simulink model "PowerSplitDriveUnit_Component_harness_model"  (R2022b)
settings: Solver=daessc  StartTime=0.0  StopTime=100  RelTol=1e-3  AbsTol=1e-3
PreLoadFcn:
  | PowerSplitDriveUnit_Component_harness_setup
undefined symbols (not defined in the file): batteryHighVoltage, Minus, Plus
libraries: fl_lib x15, nesl_utility x14, sdl_lib x2
settings Model: Creator=isaacito  LastModifiedBy=isaacito
settings SolverCC: AutoScaleAbsTol=off  AlgebraicLoopSolver=TrustRegion
settings DataIOCC: DSMLogging=off  ReturnWorkspaceOutputs=off
settings DebuggingCC: UnconnectedInputMsg=warning  UnconnectedOutputMsg=warning  UnconnectedLineMsg=warning  SymbolicDimsDataTypeCodeGenerationDiagnostic=none  SFMachineParentedDataDiag=warning
settings ModelReferenceCC: EnableRefExpFcnMdlSchedulingChecks=on
settings SFSimCC: CustomCodeUndefinedFunction=UseInterfaceOnly
settings RTWCC: DLArmComputeVersion=19.05
settings SimscapeCC: SimscapeLogType=all  SimscapeLogSimulationStatistics=on  SimscapeLogLimitData=off  SimscapeLogDataHistory=10000

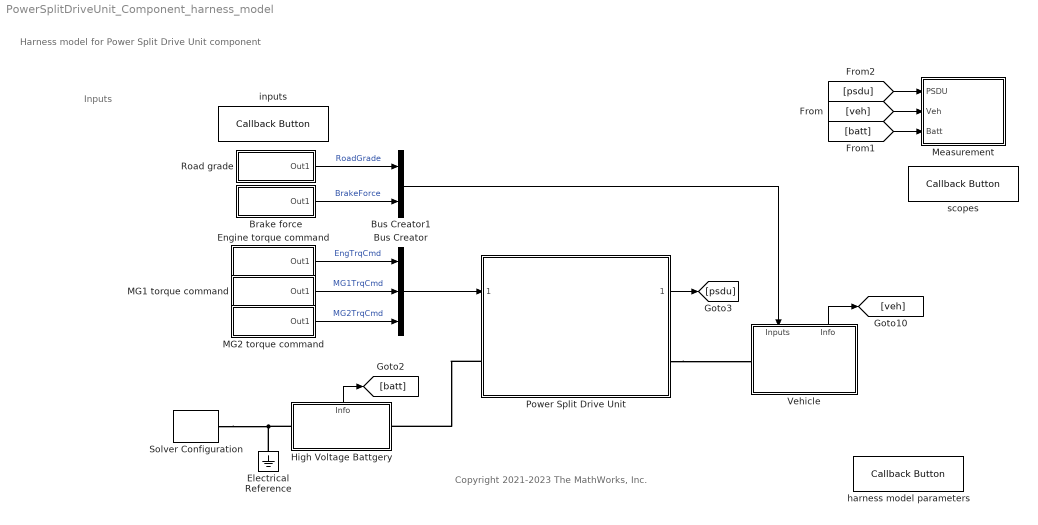
== system PowerSplitDriveUnit_Component_harness_model ==
  note: Inputs
  note: Copyright 2021-2023 The MathWorks, Inc.
  note: Harness model for Power Split Drive Unit component
  Brake force : Subsystem  mask(Continuous Multi-Step Signal){dataPoints=[0 1 0; 2 100 0], deltaT=0.1}
      mask prompts: dataPoints "Data points"; deltaT "Interpolation step [s]"
      mask help:
      | This block generates a signal consisting of smoothly connected flat segments. Data points parameter takes an N-by-3 matrix where each row specifies a flat segment. First column and second column define start and end time of the segment, respectively. Third column defines the value of the segment. Second column can also be NaN to define a point value. Flat segments and point values are smoothly interpolated by Akima spline with the specified interpolation step.
      |
      | For example, a matrix [0 1 5; 3 nan 9; 6 8 7] for Data points defines a signal as follows. First row defines a flat segment from t=0 to t=1 of value 5. Second row defines a point at t=3 of value 9. Third row defines a flat segment from t=6 to t=8 of value 7.
      mask init:
      | sig = SignalDesigner("continuous");
      | 
      | % Initialization function can access parameter names directly
      | sig.XYData = dataPoints;
      | sig.DeltaX = deltaT;
      | 
      | update(sig)
      | 
      | xStr = "[" + num2str(sig.Data.X') + "]";
      | yStr = "[" + num2str(sig.Data.Y') + "]";
      | 
      | set_param([gcb '/1-D Lookup Table'], 'Table', yStr)
      | set_param([gcb '/1-D Lookup Table'], 'BreakpointsForDimension1', xStr)
      mask DialogControl Container3 Prompt: Utility
      mask DialogControl PlotButton Prompt: Plot
      mask DialogControl PlotButton Callback:
      | dataPoints = eval(get_param(gcb, "dataPoints"));
      | deltaT = eval(get_param(gcb, "deltaT"));
      | 
      | sig = SignalDesigner("continuous");
      | sig.DeltaX = deltaT;
      | sig.XYData = dataPoints;
      | sig.XVarName = "Time (s)";
      | sig.YVarName = "Data";
      | update(sig)
      | plotDataPoints(sig);
      mask DialogControl Control3 Prompt: (invisible text area)
      mask Display: disp("Continuous" + newline + "Multi-Step")
  Bus Creator : BusCreator  Inputs=3
  Bus Creator1 : BusCreator  Inputs=2
  Electrical Reference : fl_lib/Electrical/Electrical Elements/Electrical Reference
  Engine torque command : Subsystem  mask(Continuous Multi-Step Signal){dataPoints=[0 13 0; 15 50 80; 52 100 120], deltaT=0.1}
      mask prompts: dataPoints "Data points"; deltaT "Interpolation step [s]"
      mask help:
      | This block generates a signal consisting of smoothly connected flat segments. Data points parameter takes an N-by-3 matrix where each row specifies a flat segment. First column and second column define start and end time of the segment, respectively. Third column defines the value of the segment. Second column can also be NaN to define a point value. Flat segments and point values are smoothly interpolated by Akima spline with the specified interpolation step.
      |
      | For example, a matrix [0 1 5; 3 nan 9; 6 8 7] for Data points defines a signal as follows. First row defines a flat segment from t=0 to t=1 of value 5. Second row defines a point at t=3 of value 9. Third row defines a flat segment from t=6 to t=8 of value 7.
      mask init: same as PowerSplitDriveUnit_Component_harness_model/Brake force
      mask DialogControl Container3 Prompt: Utility
      mask DialogControl PlotButton Prompt: Plot
      mask DialogControl PlotButton Callback:
      | dataPoints = eval(get_param(gcb, "dataPoints"));
      | deltaT = eval(get_param(gcb, "deltaT"));
      | 
      | sig = SignalDesigner("continuous");
      | sig.DeltaX = deltaT;
      | sig.XYData = dataPoints;
      | sig.XVarName = "Time (s)";
      | sig.YVarName = "Data";
      | update(sig)
      | plotDataPoints(sig);
      mask DialogControl Control3 Prompt: (invisible text area)
      mask Display: disp("Continuous" + newline + "Multi-Step")
  High Voltage Battgery : Subsystem
      settings: PortSchema="{\"entries\":[{\"content\":{\"sides\":[{\"content\":{\"connectorIds\":[\"LConn1\"]},\"type\":\"ConnectorPlacement.EquallySpacedRectSide\",\"uuid\":\"8acd7e9a-bb08-4de6-aa14-0989ebba81b9\"},{\"content\":{\"connectorIds\":[\"RConn1\"],\"side\":\"RIGHT\"},\"type\":\"ConnectorPlacement.EquallySpacedRectSide\",\"uuid\":\"f80e1afc-966f-4d6b-84f9-f0b60dd6f20c\"},{\"content\":{\"connectorIds\":[\"Out1\"],\"side\":\"TOP\"},\"type\":\"ConnectorPlacement.EquallySpacedRectSide\",\"uuid\":\"52ccb2b1-bd5e-4dcb-b9b6-0ef03b912c33\"}]},\"type\":\"ConnectorPlacement.EquallySpacedConnector\",\"uuid\":\"b55f48a4-f283-4a77-8513-99b31abb285a\"}],\"packageUris\":[\"http://schema.mathworks.com/mf0/Connector/R2020b\"],\"version\":\"1.0\"}"
  MG1 torque command : Subsystem  mask(Continuous Multi-Step Signal){dataPoints=[0 10 0; 12 15 9; 16 100 0], deltaT=0.1}
      mask prompts: dataPoints "Data points"; deltaT "Interpolation step [s]"
      mask help:
      | This block generates a signal consisting of smoothly connected flat segments. Data points parameter takes an N-by-3 matrix where each row specifies a flat segment. First column and second column define start and end time of the segment, respectively. Third column defines the value of the segment. Second column can also be NaN to define a point value. Flat segments and point values are smoothly interpolated by Akima spline with the specified interpolation step.
      |
      | For example, a matrix [0 1 5; 3 nan 9; 6 8 7] for Data points defines a signal as follows. First row defines a flat segment from t=0 to t=1 of value 5. Second row defines a point at t=3 of value 9. Third row defines a flat segment from t=6 to t=8 of value 7.
      mask init: same as PowerSplitDriveUnit_Component_harness_model/Brake force
      mask DialogControl Container3 Prompt: Utility
      mask DialogControl PlotButton Prompt: Plot
      mask DialogControl PlotButton Callback:
      | dataPoints = eval(get_param(gcb, "dataPoints"));
      | deltaT = eval(get_param(gcb, "deltaT"));
      | 
      | sig = SignalDesigner("continuous");
      | sig.DeltaX = deltaT;
      | sig.XYData = dataPoints;
      | sig.XVarName = "Time (s)";
      | sig.YVarName = "Data";
      | update(sig)
      | plotDataPoints(sig);
      mask DialogControl Control3 Prompt: (invisible text area)
      mask Display: disp("Continuous" + newline + "Multi-Step")
  MG2 torque command : Subsystem  mask(Continuous Multi-Step Signal){dataPoints=[0 1 0; 2 100 0], deltaT=0.1}
      mask prompts: dataPoints "Data points"; deltaT "Interpolation step [s]"
      mask help:
      | This block generates a signal consisting of smoothly connected flat segments. Data points parameter takes an N-by-3 matrix where each row specifies a flat segment. First column and second column define start and end time of the segment, respectively. Third column defines the value of the segment. Second column can also be NaN to define a point value. Flat segments and point values are smoothly interpolated by Akima spline with the specified interpolation step.
      |
      | For example, a matrix [0 1 5; 3 nan 9; 6 8 7] for Data points defines a signal as follows. First row defines a flat segment from t=0 to t=1 of value 5. Second row defines a point at t=3 of value 9. Third row defines a flat segment from t=6 to t=8 of value 7.
      mask init: same as PowerSplitDriveUnit_Component_harness_model/Brake force
      mask DialogControl Container3 Prompt: Utility
      mask DialogControl PlotButton Prompt: Plot
      mask DialogControl PlotButton Callback:
      | dataPoints = eval(get_param(gcb, "dataPoints"));
      | deltaT = eval(get_param(gcb, "deltaT"));
      | 
      | sig = SignalDesigner("continuous");
      | sig.DeltaX = deltaT;
      | sig.XYData = dataPoints;
      | sig.XVarName = "Time (s)";
      | sig.YVarName = "Data";
      | update(sig)
      | plotDataPoints(sig);
      mask DialogControl Control3 Prompt: (invisible text area)
      mask Display: disp("Continuous" + newline + "Multi-Step")
  Measurement : Subsystem
  Power Split Drive Unit : Subsystem  ReferencedSubsystem=PowerSplitDriveUnit_refsub_Basic
  Road grade : Subsystem  mask(Continuous Multi-Step Signal){dataPoints=[0 1 0; 2 100 0], deltaT=0.1}
      mask prompts: dataPoints "Data points"; deltaT "Interpolation step [s]"
      mask help:
      | This block generates a signal consisting of smoothly connected flat segments. Data points parameter takes an N-by-3 matrix where each row specifies a flat segment. First column and second column define start and end time of the segment, respectively. Third column defines the value of the segment. Second column can also be NaN to define a point value. Flat segments and point values are smoothly interpolated by Akima spline with the specified interpolation step.
      |
      | For example, a matrix [0 1 5; 3 nan 9; 6 8 7] for Data points defines a signal as follows. First row defines a flat segment from t=0 to t=1 of value 5. Second row defines a point at t=3 of value 9. Third row defines a flat segment from t=6 to t=8 of value 7.
      mask init: same as PowerSplitDriveUnit_Component_harness_model/Brake force
      mask DialogControl Container3 Prompt: Utility
      mask DialogControl PlotButton Prompt: Plot
      mask DialogControl PlotButton Callback:
      | dataPoints = eval(get_param(gcb, "dataPoints"));
      | deltaT = eval(get_param(gcb, "deltaT"));
      | 
      | sig = SignalDesigner("continuous");
      | sig.DeltaX = deltaT;
      | sig.XYData = dataPoints;
      | sig.XVarName = "Time (s)";
      | sig.YVarName = "Data";
      | update(sig)
      | plotDataPoints(sig);
      mask DialogControl Control3 Prompt: (invisible text area)
      mask Display: disp("Continuous" + newline + "Multi-Step")
  Solver Configuration : nesl_utility/Solver Configuration  PhysicalDomain=network_engine_domain  SubClassName=solver  LeftPortType=input  RightPortType=generic  Tones=[]  Harmonics=[]  SimulateNoise=off  Profile=off  UseLocalSampling=off  EnableSwitchedLinearOptims=on  FrequencyDomain=off  UseCCode=off  RelTol=0.001  AbsTol=1e-06  MinStep=1e-09  ToWorkspace=off  RevertToSquareIcSolve=off  NumHomotopyIterations=100  PhasorMode=off  PhasorModeNumHarmonics=1  ConsistencySolver=NEWTON_FTOL  IndexReductionMethod=DerivativeReplacement  DoDC=off  ResidualTolerance=1e-09  ConsistencyTolSource=GLOBAL  ConsistencyAbsTol=0.001  ConsistencyRelTol=0.001  ConsistencyTolFactor=0.001  UseLocalSolver=off  LocalSolverChoice=NE_BACKWARD_EULER_ADVANCER  ResolveIndetEquations=on  FunctionEvalNumThread=1  LocalSolverSampleTime=0.001  DoFixedCost=off  MaxNonlinIter=3  MaxModeIter=2  ComputeImpulses=off  ImpulseIterations=2  LinearAlgebra=auto  LinearAlgebraNumThread=0  EquationFormulation=NE_TIME_EF  DelaysMemoryBudget=1024  AutomaticFiltering=on  FilteringTimeConstant=0.001  PartitionStorageMethod=AS_NEEDED  PartitionMemoryBudget=1024  PartitionMethod=ROBUST
      settings: AttributesFormatString=Local solver %<UseLocalSolver>
  Vehicle : Subsystem
      settings: PortSchema="{\"entries\":[{\"content\":{\"sides\":[{\"content\":{\"connectorIds\":[\"LConn1\"]},\"type\":\"ConnectorPlacement.EquallySpacedRectSide\",\"uuid\":\"26173f4b-7c8a-4f16-9397-bd2703a262c3\"},{\"content\":{\"connectorIds\":[],\"side\":\"RIGHT\"},\"type\":\"ConnectorPlacement.EquallySpacedRectSide\",\"uuid\":\"c1cca5f5-e160-4db7-9272-a3c788f9ef94\"},{\"content\":{\"connectorIds\":[\"In1\",\"Out1\"],\"side\":\"TOP\"},\"type\":\"ConnectorPlacement.EquallySpacedRectSide\",\"uuid\":\"12b52f59-061a-44b9-b00e-a084783c45fb\"}]},\"type\":\"ConnectorPlacement.EquallySpacedConnector\",\"uuid\":\"a6613901-d795-4b91-ba16-2f1b373021b5\"}],\"packageUris\":[\"http://schema.mathworks.com/mf0/Connector/R2020b\"],\"version\":\"1.0\"}"
  harness model parameters : CallbackButton  ButtonText=Reset
      settings: ClickFcn=PowerSplitDriveUnit_Component_resetHarness
  inputs : CallbackButton  ButtonText=Plot
      settings: ClickFcn=PowerSplitDriveUnit_Component_plotInputs
  scopes : CallbackButton  ButtonText=Open
      settings: ClickFcn=|
      | open_system(bdroot + "/Measurement/Scope Harness 2")
      | 
      | % Last call appears on top.
      | open_system(bdroot + "/Measurement/Scope Harness")
  wires:
  High Voltage Battgery/1(Info) -> [batt]
  Power Split Drive Unit/1 -> [psdu]
  Vehicle/1(Info) -> [veh]
  [veh] -> Measurement/2(Veh)
  [psdu] -> Measurement/1(PSDU)
  [batt] -> Measurement/3(Batt)
  Bus Creator/1 -> Power Split Drive Unit/1
  Bus Creator1/1 -> Vehicle/1(Inputs)
  Engine torque command/1(Out1) -> Bus Creator/1  "EngTrqCmd"
  MG1 torque command/1(Out1) -> Bus Creator/2  "MG1TrqCmd"
  MG2 torque command/1(Out1) -> Bus Creator/3  "MG2TrqCmd"
  Road grade/1(Out1) -> Bus Creator1/1  "RoadGrade"
  Brake force/1(Out1) -> Bus Creator1/2  "BrakeForce"
  connections:
  High Voltage Battgery/LConn1 -- Solver Configuration/RConn1 -- Electrical Reference/LConn1
  Power Split Drive Unit/LConn1 -- High Voltage Battgery/RConn1
  Power Split Drive Unit/RConn1 -- Vehicle/LConn1

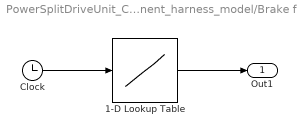
== system PowerSplitDriveUnit_Component_harness_model/Brake force ==
  1-D Lookup Table : Lookup_n-D  NumberOfTableDimensions=1  BreakpointsForDimension1="[0             1           1.1           1.2           1.3           1.4           1.5           1.6           1.7           1.8           1.9             2           100]"  Table="[0  0  0  0  0  0  0  0  0  0  0  0  0]"  InternalRulePriority=Speed  RndMeth=Simplest
  Clock : Clock
  Out1 : Outport
  wires:
  Clock/1 -> 1-D Lookup Table/1
  1-D Lookup Table/1 -> Out1/1

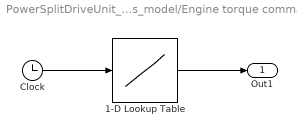
== system PowerSplitDriveUnit_Component_harness_model/Engine torque command ==
  1-D Lookup Table : Lookup_n-D  NumberOfTableDimensions=1  BreakpointsForDimension1="[0            13          13.1          13.2          13.3          13.4          13.5          13.6          13.7          13.8          13.9            14          14.1          14.2          14.3          14.4          14.5          14.6          14.7          14.8          14.9            15            50          50.1          50.2          50.3          50.4          50.5          50.6          50.7          50.8          50.9            51          51.1          51.2          51.3          51.4          51.5          51.6          51.7          51.8          51.9            52           100]"  Table="[0             0          0.58          2.24          4.86          8.32          12.5         17.28         22.54         28.16         34.02            40         45.98         51.84         57.46         62.72          67.5         71.68         75.14         77.76         79.42            80            80         80.29         81.12         82.43         84.16         86.25         88.64         91.27         94.08         97.01           100        102.99        105.92        108.73        111.36        113.75        115.84        117.57        118.88        119.71           120           120]"  InternalRulePriority=Speed  RndMeth=Simplest
  Clock : Clock
  Out1 : Outport
  wires:
  Clock/1 -> 1-D Lookup Table/1
  1-D Lookup Table/1 -> Out1/1

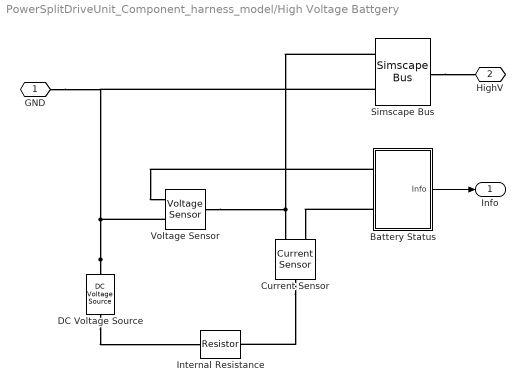
== system PowerSplitDriveUnit_Component_harness_model/High Voltage Battgery ==
  Battery Status : Subsystem
  Current Sensor : fl_lib/Electrical/Electrical Sensors/Current Sensor
  DC Voltage Source : fl_lib/Electrical/Electrical Sources/DC Voltage Source  v0=batteryHighVoltage.voltage_V V
      settings: AttributesFormatString=%<v0> [%<v0_unit>]
  Internal Resistance : fl_lib/Electrical/Electrical Elements/Resistor  R=batteryHighVoltage.internal_R_Ohm Ohm  i_specify=off  i_priority=High  i=0 A  i_nominal_specify=off  i_nominal_unit=A  i_nominal_value=1  v_specify=off  v_priority=High  v=0 V  v_nominal_specify=off  v_nominal_unit=V  v_nominal_value=1
      settings: AttributesFormatString=%<R> [%<R_unit>]
  Simscape Bus : SimscapeBus  HierarchyStrings=Plus;Minus  ConnectionType=Bus: Bus_HighVoltage
      settings: AttributesFormatString=%<ConnectionType>
  Voltage Sensor : fl_lib/Electrical/Electrical Sensors/Voltage Sensor
  GND : PMIOPort  Side=Left
  HighV : PMIOPort  Port=2  Side=Right
  Info : Outport
  wires:
  Battery Status/1(Info) -> Info/1
  connections:
  DC Voltage Source/RConn1 -- Simscape Bus/LConn2 -- GND/RConn1 -- Voltage Sensor/RConn2
  Simscape Bus/LConn1 -- Voltage Sensor/LConn1 -- Current Sensor/RConn2
  Battery Status/LConn2 -- Current Sensor/RConn1
  Simscape Bus/RConn1 -- HighV/RConn1
  Current Sensor/LConn1 -- Internal Resistance/RConn1
  DC Voltage Source/LConn1 -- Internal Resistance/LConn1
  Battery Status/LConn1 -- Voltage Sensor/RConn1

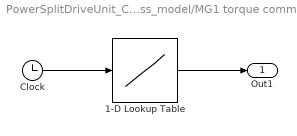
== system PowerSplitDriveUnit_Component_harness_model/MG1 torque command ==
  1-D Lookup Table : Lookup_n-D  NumberOfTableDimensions=1  BreakpointsForDimension1="[0            10          10.1          10.2          10.3          10.4          10.5          10.6          10.7          10.8          10.9            11          11.1          11.2          11.3          11.4          11.5          11.6          11.7          11.8          11.9            12            15          15.1          15.2          15.3          15.4          15.5          15.6          15.7          15.8          15.9            16           100]"  Table="[0           0     0.06525       0.252     0.54675       0.936      1.4062       1.944      2.5358       3.168      3.8273         4.5      5.1728       5.832      6.4643       7.056      7.5938       8.064      8.4533       8.748      8.9348           9           9       8.748       8.064       7.056       5.832         4.5       3.168       1.944       0.936       0.252           0           0]"  InternalRulePriority=Speed  RndMeth=Simplest
  Clock : Clock
  Out1 : Outport
  wires:
  Clock/1 -> 1-D Lookup Table/1
  1-D Lookup Table/1 -> Out1/1

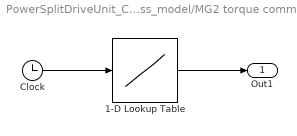
== system PowerSplitDriveUnit_Component_harness_model/MG2 torque command ==
  1-D Lookup Table : Lookup_n-D  NumberOfTableDimensions=1  BreakpointsForDimension1="[0             1           1.1           1.2           1.3           1.4           1.5           1.6           1.7           1.8           1.9             2           100]"  Table="[0  0  0  0  0  0  0  0  0  0  0  0  0]"  InternalRulePriority=Speed  RndMeth=Simplest
  Clock : Clock
  Out1 : Outport
  wires:
  Clock/1 -> 1-D Lookup Table/1
  1-D Lookup Table/1 -> Out1/1

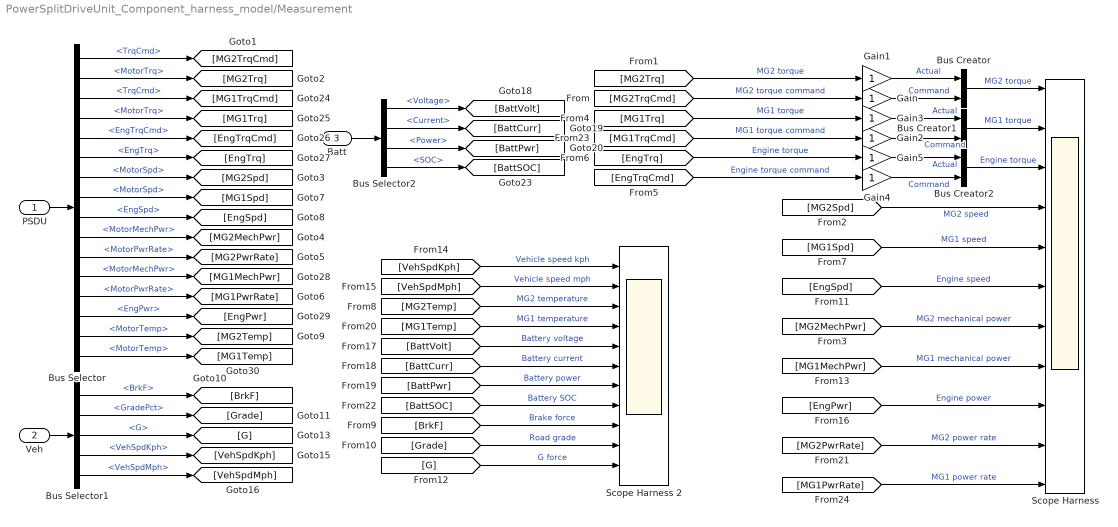
== system PowerSplitDriveUnit_Component_harness_model/Measurement ==
  PSDU : Inport
  Veh : Inport  Port=2
  Batt : Inport  Port=3
  Bus Creator : BusCreator  Inputs=2
  Bus Creator1 : BusCreator  Inputs=2
  Bus Creator2 : BusCreator  Inputs=2
  Bus Selector : BusSelector  OutputSignals=mg2.TrqCmd,mg2.MotorTrq,mg1.TrqCmd,mg1.MotorTrq,eng.EngTrqCmd,eng.EngTrq,mg2.MotorSpd,mg1.MotorSpd,eng.EngSpd,mg2.MotorMechPwr,mg2.MotorPwrRate,mg1.MotorMechPwr,mg1.MotorPwrRate,eng.EngPwr,mg2.MotorTemp,mg1.MotorTemp
  Bus Selector1 : BusSelector  OutputSignals=BrkF,GradePct,G,VehSpdKph,VehSpdMph
  Bus Selector2 : BusSelector  OutputSignals=Voltage,Current,Power,SOC
  Gain{,1..5} (6 alike) : Gain
  Scope Harness : Scope  NumInputPorts=11
  Scope Harness 2 : Scope  NumInputPorts=11
  wires:
  Veh/1 -> Bus Selector1/1
  PSDU/1 -> Bus Selector/1
  Batt/1 -> Bus Selector2/1
  Bus Selector/1 -> [MG2TrqCmd]  "<TrqCmd>"
  Bus Selector/2 -> [MG2Trq]  "<MotorTrq>"
  Bus Selector/3 -> [MG1TrqCmd]  "<TrqCmd>"
  Bus Selector/4 -> [MG1Trq]  "<MotorTrq>"
  Bus Selector/5 -> [EngTrqCmd]  "<EngTrqCmd>"
  Bus Selector/6 -> [EngTrq]  "<EngTrq>"
  Bus Selector/7 -> [MG2Spd]  "<MotorSpd>"
  Bus Selector/8 -> [MG1Spd]  "<MotorSpd>"
  Bus Selector/9 -> [EngSpd]  "<EngSpd>"
  Bus Selector/10 -> [MG2MechPwr]  "<MotorMechPwr>"
  Bus Selector/12 -> [MG1MechPwr]  "<MotorMechPwr>"
  Bus Selector/14 -> [EngPwr]  "<EngPwr>"
  Bus Selector/15 -> [MG2Temp]  "<MotorTemp>"
  Bus Selector/16 -> [MG1Temp]  "<MotorTemp>"
  Bus Selector1/1 -> [BrkF]  "<BrkF>"
  Bus Selector1/2 -> [Grade]  "<GradePct>"
  Bus Selector1/3 -> [G]  "<G>"
  Bus Selector1/4 -> [VehSpdKph]  "<VehSpdKph>"
  Bus Selector1/5 -> [VehSpdMph]  "<VehSpdMph>"
  Bus Selector2/1 -> [BattVolt]  "<Voltage>"
  Bus Selector2/2 -> [BattCurr]  "<Current>"
  Bus Selector2/3 -> [BattPwr]  "<Power>"
  Bus Selector2/4 -> [BattSOC]  "<SOC>"
  [MG2TrqCmd] -> Gain/1  "MG2 torque command"
  [MG2Trq] -> Gain1/1  "MG2 torque"
  [MG1TrqCmd] -> Gain2/1  "MG1 torque command"
  [MG1Trq] -> Gain3/1  "MG1 torque"
  [EngTrqCmd] -> Gain4/1  "Engine torque command"
  [EngTrq] -> Gain5/1  "Engine torque"
  Bus Creator/1 -> Scope Harness/1  "MG2 torque"
  Bus Creator1/1 -> Scope Harness/2  "MG1 torque"
  Bus Creator2/1 -> Scope Harness/3  "Engine torque"
  [MG2Spd] -> Scope Harness/4  "MG2 speed"
  [MG1Spd] -> Scope Harness/5  "MG1 speed"
  [EngSpd] -> Scope Harness/6  "Engine speed"
  [MG2MechPwr] -> Scope Harness/7  "MG2 mechanical power"
  [MG1MechPwr] -> Scope Harness/8  "MG1 mechanical power"
  [EngPwr] -> Scope Harness/9  "Engine power"
  [VehSpdKph] -> Scope Harness 2/1  "Vehicle speed kph"
  [VehSpdMph] -> Scope Harness 2/2  "Vehicle speed mph"
  [MG2Temp] -> Scope Harness 2/3  "MG2 temperature"
  [MG1Temp] -> Scope Harness 2/4  "MG1 temperature"
  [BattVolt] -> Scope Harness 2/5  "Battery voltage"
  [BattCurr] -> Scope Harness 2/6  "Battery current"
  [BattPwr] -> Scope Harness 2/7  "Battery power"
  [BattSOC] -> Scope Harness 2/8  "Battery SOC"
  [BrkF] -> Scope Harness 2/9  "Brake force"
  [Grade] -> Scope Harness 2/10  "Road grade"
  [G] -> Scope Harness 2/11  "G force"
  Bus Selector/11 -> [MG2PwrRate]  "<MotorPwrRate>"
  Bus Selector/13 -> [MG1PwrRate]  "<MotorPwrRate>"
  [MG2PwrRate] -> Scope Harness/10  "MG2 power rate"
  [MG1PwrRate] -> Scope Harness/11  "MG1 power rate"
  Gain1/1 -> Bus Creator/1  "Actual"
  Gain/1 -> Bus Creator/2  "Command"
  Gain3/1 -> Bus Creator1/1  "Actual"
  Gain2/1 -> Bus Creator1/2  "Command"
  Gain5/1 -> Bus Creator2/1  "Actual"
  Gain4/1 -> Bus Creator2/2  "Command"

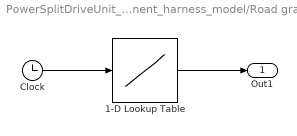
== system PowerSplitDriveUnit_Component_harness_model/Road grade ==
  1-D Lookup Table : Lookup_n-D  NumberOfTableDimensions=1  BreakpointsForDimension1="[0             1           1.1           1.2           1.3           1.4           1.5           1.6           1.7           1.8           1.9             2           100]"  Table="[0  0  0  0  0  0  0  0  0  0  0  0  0]"  InternalRulePriority=Speed  RndMeth=Simplest
  Clock : Clock
  Out1 : Outport
  wires:
  Clock/1 -> 1-D Lookup Table/1
  1-D Lookup Table/1 -> Out1/1

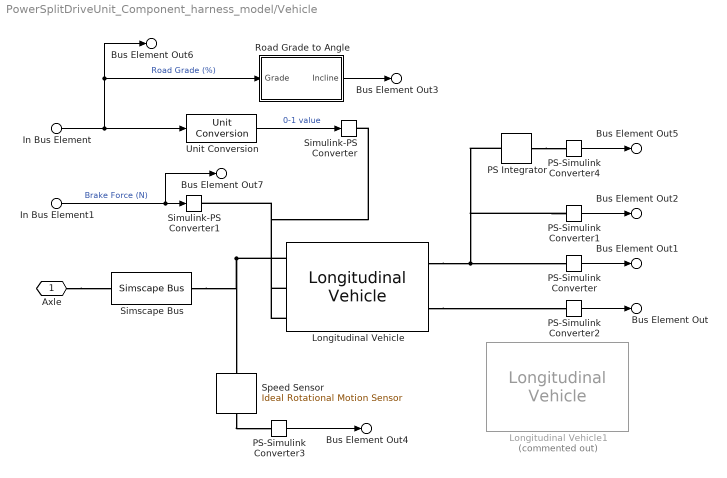
== system PowerSplitDriveUnit_Component_harness_model/Vehicle ==
  In Bus Element : Inport  PortName=Inputs  Element=RoadGrade
      settings: AttributesFormatString=%<Unit>
  In Bus Element1 : Inport  PortName=Inputs  Element=BrakeForce
      settings: AttributesFormatString=%<Unit>
  Longitudinal Vehicle : sdl_lib/Tires & Vehicles/Longitudinal Vehicle  vehParamType=sdl.enum.VehicleParameterizationType.RoadLoad  M_vehicle=1550 kg  R_tireroll=0.3 m  C_tireroll=0.0136  C_airdrag=0.25  A_front=2.4 m^2  A_rl=175 N  B_rl=0 N/(m/s)  C_rl=0.032 N/(km/hr)^2  g=9.81 m/s^2  V_1=1 kph  w_1=1 rpm  ShowBrakeIn=simscape.enum.onoff.on  ShowSlopeIn=simscape.enum.onoff.on  SlopeInputType=sdl.enum.VehicleLongitudinalRoadSlopeInputType.Grade  ShowWindIn=simscape.enum.onoff.off  ShowGOut=simscape.enum.onoff.on  air_density=1.184 kg/m^3  V_x_specify=on  V_x_priority=High  V_x=initial.vehicle_speed_kph km/hr  V_x_nominal_specify=off  V_x_nominal_unit=m/s  V_x_nominal_value=1  trq_specify=off  trq_priority=None  trq=0 N*m  trq_nominal_specify=off  trq_nominal_unit=N*m  trq_nominal_value=1  w_specify=off  w_priority=None  w=0 rad/s  w_nominal_specify=off  w_nominal_unit=rad/s  w_nominal_value=1
      settings: InternalSimscapePortConfiguration="{\"Bottom\":[],\"Left\":[{\"id\":\"Axle\",\"label\":\"Axle\",\"type\":\"foundation.mechanical.rotational.rotational\"}],\"Right\":[{\"id\":\"v_out\",\"label\":\"VehSpd\",\"type\":\"output\"},{\"id\":\"G_out\",\"label\":\"G\",\"type\":\"output\"}],\"Top\":[{\"id\":\"brkF\",\"label\":\"Brake\",\"type\":\"input\"},{\"id\":\"grade_norm\",\"label\":\"NG\",\"type\":\"input\"}]}"
      settings: AttributesFormatString=|
      | %<V_x> [%<V_x_unit>]
      | Priority: %<V_x_priority>
  Longitudinal Vehicle1 : sdl_lib/Tires & Vehicles/Longitudinal Vehicle  Commented=on  vehParamType=sdl.enum.VehicleParameterizationType.Regular  M_vehicle=1550 kg  R_tireroll=0.3 m  C_tireroll=0.0136  C_airdrag=0.25  A_front=2.4 m^2  A_rl=120 N  B_rl=1.8 N/(m/s)  C_rl=0.389 N/(m/s)^2  g=9.81 m/s^2  V_1=1 kph  w_1=1 rpm  ShowBrakeIn=simscape.enum.onoff.on  ShowSlopeIn=simscape.enum.onoff.on  SlopeInputType=sdl.enum.VehicleLongitudinalRoadSlopeInputType.Grade  ShowWindIn=simscape.enum.onoff.off  ShowGOut=simscape.enum.onoff.on  air_density=1.184 kg/m^3  V_x_specify=on  V_x_priority=High  V_x=initial.vehicle_speed_kph km/hr  V_x_nominal_specify=off  V_x_nominal_unit=m/s  V_x_nominal_value=1  trq_specify=off  trq_priority=None  trq=0 N*m  trq_nominal_specify=off  trq_nominal_unit=N*m  trq_nominal_value=1  w_specify=off  w_priority=None  w=0 rad/s  w_nominal_specify=off  w_nominal_unit=rad/s  w_nominal_value=1
      settings: InternalSimscapePortConfiguration="{\"Bottom\":[],\"Left\":[{\"id\":\"Axle\",\"label\":\"Axle\",\"type\":\"foundation.mechanical.rotational.rotational\"}],\"Right\":[{\"id\":\"v_out\",\"label\":\"VehSpd\",\"type\":\"output\"},{\"id\":\"G_out\",\"label\":\"G\",\"type\":\"output\"}],\"Top\":[{\"id\":\"brkF\",\"label\":\"Brake\",\"type\":\"input\"},{\"id\":\"grade_norm\",\"label\":\"NG\",\"type\":\"input\"}]}"
      settings: AttributesFormatString=|
      | %<V_x> [%<V_x_unit>]
      | Priority: %<V_x_priority>
  PS Integrator : fl_lib/Physical Signals/Linear Operators/PS Integrator  reset_method=foundation.enum.IntegratorResetSpec.None  initial_condition_spec=foundation.enum.IntegratorICSpec.Internal  saturation_spec=foundation.enum.IntegratorSaturationSpec.None  saturation_source_spec=foundation.enum.IntegratorSaturationSourceSpec.Internal  x0=0 km  xu=inf s  xl=-inf s
      settings: AttributesFormatString=Initial: %<x0> %<x0_unit>
  PS-Simulink Converter : nesl_utility/PS-Simulink Converter  PhysicalDomain=network_engine_domain  SubClassName=ps_output  LeftPortType=input  RightPortType=output  PseudoPeriodic=off  Frequencies=[]  VectorFormat=1-D array  Unit=km/hr  AffineConversion=off
  PS-Simulink Converter1 : nesl_utility/PS-Simulink Converter  PhysicalDomain=network_engine_domain  SubClassName=ps_output  LeftPortType=input  RightPortType=output  PseudoPeriodic=off  Frequencies=[]  VectorFormat=1-D array  Unit=mph  AffineConversion=off
  PS-Simulink Converter2 : nesl_utility/PS-Simulink Converter  PhysicalDomain=network_engine_domain  SubClassName=ps_output  LeftPortType=input  RightPortType=output  PseudoPeriodic=off  Frequencies=[]  VectorFormat=1-D array  Unit=1  AffineConversion=off
  PS-Simulink Converter3 : nesl_utility/PS-Simulink Converter  PhysicalDomain=network_engine_domain  SubClassName=ps_output  LeftPortType=input  RightPortType=output  PseudoPeriodic=off  Frequencies=[]  VectorFormat=1-D array  Unit=rpm  AffineConversion=off
  PS-Simulink Converter4 : nesl_utility/PS-Simulink Converter  PhysicalDomain=network_engine_domain  SubClassName=ps_output  LeftPortType=input  RightPortType=output  PseudoPeriodic=off  Frequencies=[]  VectorFormat=1-D array  Unit=km  AffineConversion=off
  Road Grade to Angle : Subsystem
  Simscape Bus : SimscapeBus  HierarchyStrings=AngSpd  ConnectionType=Bus: Bus_Rotational
      settings: AttributesFormatString=%<ConnectionType>
  Simulink-PS Converter : nesl_utility/Simulink-PS Converter  PhysicalDomain=network_engine_domain  SubClassName=ps_input  LeftPortType=input  RightPortType=output  PseudoPeriodic=off  Frequencies=[]  NoiseDistribution=none  NoiseParameters=[]  Unit=1  AffineConversion=off  FilteringAndDerivatives=filter  SimscapeFilterOrder=1  InputFilterTimeConstant=0.001  UdotUserProvided=0
  Simulink-PS Converter1 : nesl_utility/Simulink-PS Converter  PhysicalDomain=network_engine_domain  SubClassName=ps_input  LeftPortType=input  RightPortType=output  PseudoPeriodic=off  Frequencies=[]  NoiseDistribution=none  NoiseParameters=[]  Unit=N  AffineConversion=off  FilteringAndDerivatives=filter  SimscapeFilterOrder=1  InputFilterTimeConstant=0.001  UdotUserProvided=0
  Speed Sensor : fl_lib/Mechanical/Mechanical Sensors/Ideal Rotational Motion Sensor  reference=foundation.enum.MeasurementReference.absolute  acceleration_port=false  velocity_port=true  position_port=false  wrap_angle=simscape.enum.onoff.off  offset=0 rad
      settings: InternalSimscapePortConfiguration="{\"Bottom\":[],\"Left\":[{\"id\":\"R\",\"label\":\"R\",\"type\":\"foundation.mechanical.rotational.rotational\"}],\"Right\":[{\"id\":\"W\",\"label\":\"W\",\"type\":\"output\"}],\"Top\":[]}"
  Unit Conversion : UnitConversion  OutputType=Inherit: Inherit via back propagation
  Axle : PMIOPort  Side=Left
  Bus Element Out : Outport  PortName=Info  Element=G
      settings: AttributesFormatString=%<Unit>
  Bus Element Out1 : Outport  PortName=Info  Element=VehSpdKph
      settings: AttributesFormatString=%<Unit>
  Bus Element Out2 : Outport  PortName=Info  Element=VehSpdMph
      settings: AttributesFormatString=%<Unit>
  Bus Element Out3 : Outport  PortName=Info  Element=InclineDeg
      settings: AttributesFormatString=%<Unit>
  Bus Element Out4 : Outport  PortName=Info  Element=AxleSpd
      settings: AttributesFormatString=%<Unit>
  Bus Element Out5 : Outport  PortName=Info  Element=TavelDist
      settings: AttributesFormatString=%<Unit>
  Bus Element Out6 : Outport  PortName=Info  Element=GradePct
      settings: AttributesFormatString=%<Unit>
  Bus Element Out7 : Outport  PortName=Info  Element=BrkF
      settings: AttributesFormatString=%<Unit>
  wires:
  PS-Simulink Converter1/1 -> Bus Element Out2/1
  Unit Conversion/1 -> Simulink-PS Converter/1  "0-1 value"
  In Bus Element1/1 -> Bus Element Out7/1, Simulink-PS Converter1/1  "Brake Force (N)"
  PS-Simulink Converter3/1 -> Bus Element Out4/1
  PS-Simulink Converter/1 -> Bus Element Out1/1
  In Bus Element/1 -> Bus Element Out6/1, Road Grade to Angle/1(Grade), Unit Conversion/1  "Road Grade (%)"
  PS-Simulink Converter2/1 -> Bus Element Out/1
  Road Grade to Angle/1(Incline) -> Bus Element Out3/1
  PS-Simulink Converter4/1 -> Bus Element Out5/1
  connections:
  Longitudinal Vehicle/RConn1 -- PS Integrator/LConn1 -- PS-Simulink Converter1/LConn1 -- PS-Simulink Converter/LConn1
  Longitudinal Vehicle/LConn2 -- Simulink-PS Converter1/RConn1
  Longitudinal Vehicle/LConn3 -- Simulink-PS Converter/RConn1
  Speed Sensor/RConn1 -- PS-Simulink Converter3/LConn1
  Longitudinal Vehicle/RConn2 -- PS-Simulink Converter2/LConn1
  Longitudinal Vehicle/LConn1 -- Simscape Bus/LConn1 -- Speed Sensor/LConn1
  Axle/RConn1 -- Simscape Bus/RConn1
  PS Integrator/RConn1 -- PS-Simulink Converter4/LConn1

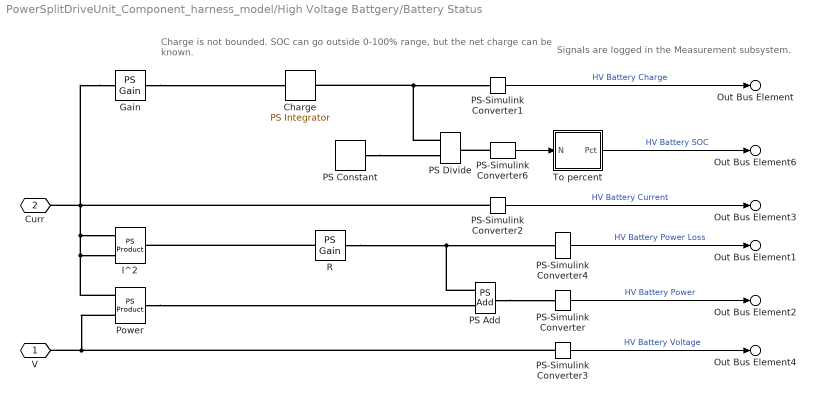
== system PowerSplitDriveUnit_Component_harness_model/High Voltage Battgery/Battery Status ==
  note: Signals are logged in the Measurement subsystem.
  note: Charge is not bounded. SOC can go outside 0-100% range,
      | but the net charge can be known.
  Charge : fl_lib/Physical Signals/Linear Operators/PS Integrator  reset_method=foundation.enum.IntegratorResetSpec.None  initial_condition_spec=foundation.enum.IntegratorICSpec.Internal  saturation_spec=foundation.enum.IntegratorSaturationSpec.None  saturation_source_spec=foundation.enum.IntegratorSaturationSourceSpec.Internal  x0=initial.hvBattery_Charge_Ahr A*hr  xu=inf s  xl=-inf s
      settings: AttributesFormatString=%<x0> [%<x0_unit>]
  Gain : fl_lib/Physical Signals/Functions/PS Gain  gain=-1
      settings: AttributesFormatString=%<gain>
  I^2 : fl_lib/Physical Signals/Functions/PS Product
  PS Add : fl_lib/Physical Signals/Functions/PS Add
  PS Constant : fl_lib/Physical Signals/Sources/PS Constant  constant=batteryHighVoltage.charge_Ahr A*hr
      settings: AttributesFormatString=%<constant> [%<constant_unit>]
  PS Divide : fl_lib/Physical Signals/Functions/PS Divide
  PS-Simulink Converter : nesl_utility/PS-Simulink Converter  PhysicalDomain=network_engine_domain  SubClassName=ps_output  LeftPortType=input  RightPortType=output  PseudoPeriodic=off  Frequencies=[]  VectorFormat=1-D array  Unit=kW  AffineConversion=off
  PS-Simulink Converter1 : nesl_utility/PS-Simulink Converter  PhysicalDomain=network_engine_domain  SubClassName=ps_output  LeftPortType=input  RightPortType=output  PseudoPeriodic=off  Frequencies=[]  VectorFormat=1-D array  Unit=A*hr  AffineConversion=off
  PS-Simulink Converter2 : nesl_utility/PS-Simulink Converter  PhysicalDomain=network_engine_domain  SubClassName=ps_output  LeftPortType=input  RightPortType=output  PseudoPeriodic=off  Frequencies=[]  VectorFormat=1-D array  Unit=A  AffineConversion=off
  PS-Simulink Converter3 : nesl_utility/PS-Simulink Converter  PhysicalDomain=network_engine_domain  SubClassName=ps_output  LeftPortType=input  RightPortType=output  PseudoPeriodic=off  Frequencies=[]  VectorFormat=1-D array  Unit=V  AffineConversion=off
  PS-Simulink Converter4 : nesl_utility/PS-Simulink Converter  PhysicalDomain=network_engine_domain  SubClassName=ps_output  LeftPortType=input  RightPortType=output  PseudoPeriodic=off  Frequencies=[]  VectorFormat=1-D array  Unit=W  AffineConversion=off
  PS-Simulink Converter6 : nesl_utility/PS-Simulink Converter  PhysicalDomain=network_engine_domain  SubClassName=ps_output  LeftPortType=input  RightPortType=output  PseudoPeriodic=off  Frequencies=[]  VectorFormat=1-D array  Unit=1  AffineConversion=off
  Power : fl_lib/Physical Signals/Functions/PS Product
  R : fl_lib/Physical Signals/Functions/PS Gain  gain=batteryHighVoltage.internal_R_Ohm Ohm
      settings: AttributesFormatString=%<gain> [%<gain_unit>]
  To percent : Subsystem
  V : PMIOPort  Side=Left
  Curr : PMIOPort  Port=2  Side=Left
  Out Bus Element : Outport  PortName=Info  Element=Charge
      settings: AttributesFormatString=%<Unit>
  Out Bus Element3 : Outport  PortName=Info  Element=Current
      settings: AttributesFormatString=%<Unit>
  Out Bus Element1 : Outport  PortName=Info  Element=PowerLoss
      settings: AttributesFormatString=%<Unit>
  Out Bus Element2 : Outport  PortName=Info  Element=Power
      settings: AttributesFormatString=%<Unit>
  Out Bus Element4 : Outport  PortName=Info  Element=Voltage
      settings: AttributesFormatString=%<Unit>
  Out Bus Element6 : Outport  PortName=Info  Element=SOC
      settings: AttributesFormatString=%<Unit>
  wires:
  PS-Simulink Converter6/1 -> To percent/1(N)
  To percent/1(Pct) -> Out Bus Element6/1  "HV Battery SOC"
  PS-Simulink Converter3/1 -> Out Bus Element4/1  "HV Battery Voltage"
  PS-Simulink Converter2/1 -> Out Bus Element3/1  "HV Battery Current"
  PS-Simulink Converter4/1 -> Out Bus Element1/1  "HV Battery Power Loss"
  PS-Simulink Converter1/1 -> Out Bus Element/1  "HV Battery Charge"
  PS-Simulink Converter/1 -> Out Bus Element2/1  "HV Battery Power"
  connections:
  PS-Simulink Converter6/LConn1 -- PS Divide/RConn1
  Power/RConn1 -- PS Add/LConn2
  PS Constant/RConn1 -- PS Divide/LConn2
  PS Add/RConn1 -- PS-Simulink Converter/LConn1
  R/LConn1 -- I^2/RConn1
  PS Divide/LConn1 -- PS-Simulink Converter1/LConn1 -- Charge/RConn1
  Gain/RConn1 -- Charge/LConn1
  PS Add/LConn1 -- PS-Simulink Converter4/LConn1 -- R/RConn1
  Power/LConn1 -- PS-Simulink Converter3/LConn1 -- V/RConn1
  Gain/LConn1 -- PS-Simulink Converter2/LConn1 -- Curr/RConn1 -- I^2/LConn1 -- Power/LConn2 -- I^2/LConn2

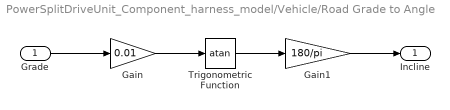
== system PowerSplitDriveUnit_Component_harness_model/Vehicle/Road Grade to Angle ==
  Grade : Inport  Unit=%
      settings: AttributesFormatString=%<Unit>
  Gain : Gain  Gain=0.01
  Gain1 : Gain  Gain=180/pi
  Trigonometric Function : Trigonometry  Operator=atan
  Incline : Outport  Unit=deg
      settings: AttributesFormatString=%<Unit>
  wires:
  Gain/1 -> Trigonometric Function/1
  Grade/1 -> Gain/1
  Trigonometric Function/1 -> Gain1/1
  Gain1/1 -> Incline/1

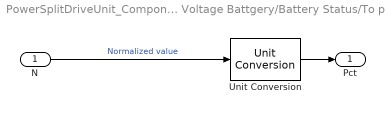
== system PowerSplitDriveUnit_Component_harness_model/High Voltage Battgery/Battery Status/To percent ==
  N : Inport
  Unit Conversion : UnitConversion
  Pct : Outport  Unit=%
      settings: AttributesFormatString=%<Unit>
  wires:
  N/1 -> Unit Conversion/1  "Normalized value"
  Unit Conversion/1 -> Pct/1
